simulink model "model_dyskretny_1_2"  (R2020a)
settings: Solver=VariableStepAuto  StartTime=0.0  StopTime=5  RelTol=1e-3
values from neighbouring files (symbols this model uses):
  ic = 0.0    (= 0)    [pom.m]    (also in zad1_4.m = 0.01)
  T = 0.5    [pom.m]    (also in zad1_10.m; zad1_4.m; zad1_6_1.m; zad1_6_2.m)
settings Model: Creator=jakub  LastModifiedBy=jakub

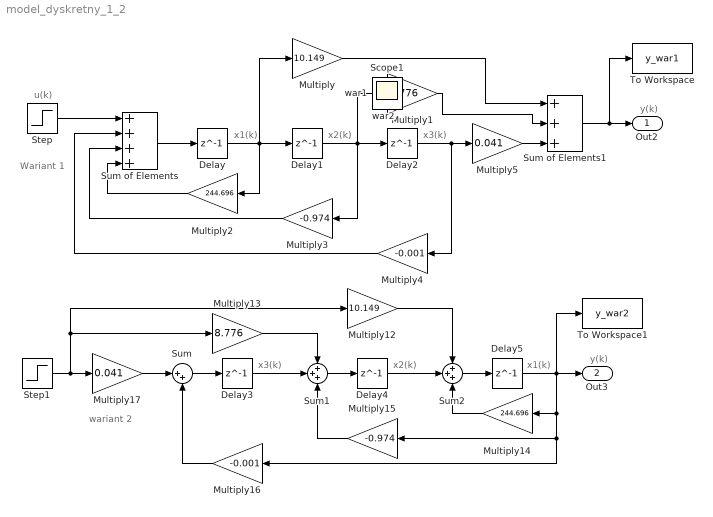
== system model_dyskretny_1_2 ==
  note: Wariant 1
  note: wariant 2
  note: x1(k)
  note: u(k)
  note: x2(k)
  note: x3(k)
  note: y(k)
  note: x2(k)
  note: y(k)
  note: x1(k)
  note: x3(k)
  Delay{,1..5} (6 alike) : Delay  DelayLength=1  InitialCondition=ic  SampleTime=T
  Multiply : Gain  Gain=10.149
  Multiply1 : Gain  Gain=8.776
  Multiply12 : Gain  Gain=10.149
  Multiply13 : Gain  Gain=8.776
  Multiply14 : Gain  Gain=244.696
  Multiply15 : Gain  Gain=-0.974
  Multiply16 : Gain  Gain=-0.001
  Multiply17 : Gain  Gain=0.041
  Multiply2 : Gain  Gain=244.696
  Multiply3 : Gain  Gain=-0.974
  Multiply4 : Gain  Gain=-0.001
  Multiply5 : Gain  Gain=0.041
  Step : Step  SampleTime=0
  Step1 : Step  SampleTime=0
  Sum : Sum  Inputs=|++
  Sum of Elements : Sum  Inputs=++++
  Sum of Elements1 : Sum  Inputs=+++
  Sum1 : Sum  Inputs=+++
  Sum2 : Sum  Inputs=+++
  To Workspace : ToWorkspace  VariableName=y_war1  SaveFormat=Structure With Time  SampleTime=T
  To Workspace1 : ToWorkspace  VariableName=y_war2  SaveFormat=Structure With Time  SampleTime=T
  Out2 : Outport
  Out3 : Outport  Port=2
  Scope1 : Scope
  war1 : Scope
  war2 : Scope
  wires:
  Step/1 -> Sum of Elements/1
  Delay/1 -> Multiply2/1, Multiply/1, Delay1/1
  Sum of Elements/1 -> Delay/1
  Delay1/1 -> Multiply1/1, Multiply3/1, Delay2/1
  Delay2/1 -> Multiply4/1, Multiply5/1
  Multiply2/1 -> Sum of Elements/4
  Multiply5/1 -> Sum of Elements1/3
  Multiply3/1 -> Sum of Elements/3
  Multiply4/1 -> Sum of Elements/2
  Multiply1/1 -> Sum of Elements1/2
  Multiply/1 -> Sum of Elements1/1
  Sum of Elements1/1 -> To Workspace/1, Out2/1
  Multiply16/1 -> Sum/2
  Multiply17/1 -> Sum/1
  Multiply14/1 -> Sum2/3
  Delay4/1 -> Sum2/2
  Sum/1 -> Delay3/1
  Sum1/1 -> Delay4/1
  Multiply15/1 -> Sum1/3
  Step1/1 -> Multiply17/1, Multiply12/1, Multiply13/1
  Multiply13/1 -> Sum1/1
  Sum2/1 -> Delay5/1
  Multiply12/1 -> Sum2/1
  Delay3/1 -> Sum1/2
  Delay5/1 -> To Workspace1/1, Multiply16/1, Multiply15/1, Multiply14/1, Out3/1
